simulink model "FourthCOMController"  (Simulink 7.9)
settings: Solver=ode3  StartTime=0.0  StopTime=inf  RelTol=1e-3
libraries: WBCLibrary x10, dspmtrx3 x4, simulink x4, simulink_extras x1
settings Model: Creator=jorhabib  LastModifiedBy=daniele
settings CustomProperty: DataType=string  Value=0

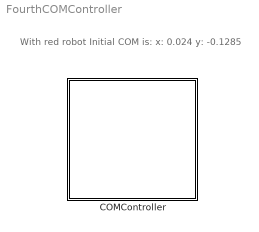
== system FourthCOMController ==
  note: With red robot Initial COM is:
      | x:  0.024
      | y:  -0.1285
  COMController : Subsystem  mask{robotName='icubSim', Ts=0.01}
      mask prompts: robotName "Robot Name"; Ts "Rate (sec)"

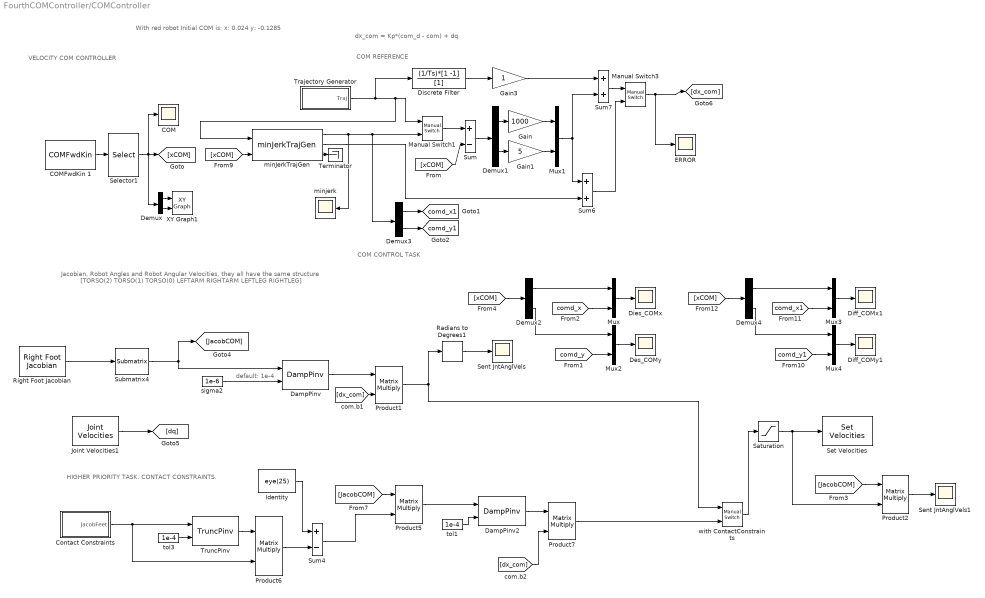
== system FourthCOMController/COMController ==
  note: COM CONTROL TASK
  note: VELOCITY COM CONTROLLER
  note: dx_com = Kp*(com_d - com) + dq
  note: default: 1e-4
  note: Jacobian, Robot Angles and Robot Angular Velocities, they all have the same structure
      | [TORSO(2)  TORSO(1)  TORSO(0)    LEFTARM    RIGHTARM    LEFTLEG    RIGHTLEG]
  note: COM REFERENCE
  note: HIGHER PRIORITY TASK. CONTACT CONSTRAINTS.
  note: With red robot Initial COM is:
      | x:  0.024
      | y:  -0.1285
  COM : Scope
      settings: TimeRange=100  YMin=-0.1  YMax=0.175  SaveName=ScopeData4
  COMFwdKin 1 : WBCLibrary/wholeBodyModel/Forward Kinematics/COMFwdKin   robotName=robotName  localName=localName
  Contact Constraints : Subsystem
  DampPinv : WBCLibrary/Utilities/DampPinv  tol=1e-4
  DampPinv2 : WBCLibrary/Utilities/DampPinv  tol=1e-4
  Demux{,1..4} (5 alike) : Demux  Outputs=2
  Des_COMy : Scope
      settings: TimeRange=100  YMin=-0.1425  YMax=-0.1125  SaveName=ScopeData6
  Dies_COMx : Scope
      settings: TimeRange=100  YMin=0.01  YMax=0.04  SaveName=ScopeData2
  Diff_COMx1 : Scope
      settings: TimeRange=100  YMin=0.0215  YMax=0.03  SaveName=ScopeData5
  Diff_COMy1 : Scope
      settings: TimeRange=100  YMin=-0.135  YMax=-0.0925  SaveName=ScopeData7
  Discrete Filter : DiscreteFilter  Numerator=(1/Ts)*[1 -1]  Denominator=[1]
  ERROR : Scope
      settings: TimeRange=100  YMin=-0.015  YMax=0.015  SaveName=ScopeData3
  Gain : Gain  Gain=1000
  Gain1 : Gain  Gain=5
  Gain3 : Gain
  Identity : Constant  Value=eye(25)
  Joint Velocities1 : WBCLibrary/wholeBodyStates/Joint Velocities  robotName=robotName  localName=localName
  Manual Switch1 : simulink/Signal Routing/Manual Switch  sw=1  action=0  varsize=off
  Manual Switch3 : simulink/Signal Routing/Manual Switch  sw=1  action=0  varsize=off
  Mux{,1..4} (5 alike) : Mux  Inputs=2
  Product{1..2,5..7} (5 alike) : Product  Multiplication=Matrix(*)  RndMeth=Zero
  Radians to Degrees1 : simulink_extras/Transformations/Radians to Degrees
  Right Foot Jacobian : WBCLibrary/wholeBodyModel/Jacobians/Right Foot Jacobian  robotName=robotName  localName=localName
  Saturation : Saturate  UpperLimit=0.8  LowerLimit=-0.8
  Selector1 : Selector  IndexMode=Zero-based  InputPortWidth=7  IndexOptions=Index vector (dialog)  Indices=[0:1]  OutputSizes=1
  Sent JntAnglVels : Scope
      settings: YMin=-0.04  YMax=0.03
  Sent JntAnglVels1 : Scope
      settings: TimeRange=100  YMin=-0.01  YMax=0.01  SaveName=ScopeData8
  Set Velocities : WBCLibrary/wholeBodyActuators/Set Velocities  val=4  robotName=robotName  localName=localName
  Submatrix4 : dspmtrx3/Submatrix  RowSpan=Range of rows  RowStartMode=First  RowStartIndex=1  RowEndMode=Index  RowEndIndex=2  ColSpan=Range of columns  ColStartMode=Index  ColStartIndex=7  ColEndMode=Last  ColEndIndex=6
  Sum : Sum  Inputs=+-
  Sum4 : Sum  Inputs=+-
  Sum6 : Sum
  Sum7 : Sum
  Terminator : Terminator
  Trajectory Generator : Subsystem
  TruncPinv : WBCLibrary/Utilities/TruncPinv  tol=1e-4
  XY Graph1 : simulink/Sinks/XY Graph  xmin=0.01  xmax=0.04  ymin=-0.15  ymax=-0.115  st=-1
  minJerkTrajGen : WBCLibrary/Utilities/minJerkTrajGen  dim=3  Ts=Ts  Tt=Tt
  minjerk : Scope
      settings: TimeRange=100  YMin=-0.12  YMax=-0.025
  sigma2 : Constant  Value=1e-6
  tol1 : Constant  Value=1e-4
  tol3 : Constant  Value=1e-4
  with ContactConstraints : simulink/Signal Routing/Manual Switch  sw=1  action=0  varsize=off
  tag scope: comd_x1=global, comd_y1=global
  wires:
  [xCOM] -> Sum/2
  Sum/1 -> Demux1/1
  Selector1/1 -> [xCOM], Demux/1, COM/1
  COMFwdKin 1/1 -> Selector1/1
  sigma2/1 -> DampPinv/2
  Submatrix4/1 -> DampPinv/1, [JacobCOM]
  [dx_com] -> Product1/2
  Product1/1 -> Radians to Degrees1/1, with ContactConstraints/1
  Radians to Degrees1/1 -> Sent JntAnglVels/1
  Demux/1 -> XY Graph1/1
  Demux/2 -> XY Graph1/2
  Mux/1 -> Dies_COMx/1
  [comd_x] -> Mux/2
  Demux1/1 -> Gain/1
  Demux1/2 -> Gain1/1
  Gain/1 -> Mux1/1
  Gain1/1 -> Mux1/2
  [comd_y] -> Mux2/2
  Mux2/1 -> Des_COMy/1
  [xCOM] -> Demux2/1
  Demux2/1 -> Mux/1
  Demux2/2 -> Mux2/1
  Right Foot Jacobian/1 -> Submatrix4/1
  [JacobCOM] -> Product5/1
  Identity/1 -> Sum4/1
  tol3/1 -> TruncPinv/2
  TruncPinv/1 -> Product6/1
  Product6/1 -> Sum4/2
  Contact Constraints/1(JacobFeet) -> TruncPinv/1, Product6/2
  Sum4/1 -> Product5/2
  Product5/1 -> DampPinv2/1
  tol1/1 -> DampPinv2/2
  [dx_com] -> Product7/2
  Product7/1 -> with ContactConstraints/2
  with ContactConstraints/1 -> Saturation/1
  Manual Switch1/1 -> Sum/1
  Trajectory Generator/1(Traj) -> minJerkTrajGen/1, Manual Switch1/1, Discrete Filter/1
  [xCOM] -> minJerkTrajGen/2
  minJerkTrajGen/1 -> minjerk/1, Manual Switch1/2, Demux3/1
  Mux1/1 -> Sum6/1, Sum7/2
  Sum6/1 -> Manual Switch3/2
  minJerkTrajGen/2 -> Sum6/2
  Demux3/1 -> [comd_x1]
  Demux3/2 -> [comd_y1]
  Mux3/1 -> Diff_COMx1/1
  [comd_x1] -> Mux3/2
  [comd_y1] -> Mux4/2
  Mux4/1 -> Diff_COMy1/1
  [xCOM] -> Demux4/1
  Demux4/1 -> Mux3/1
  Demux4/2 -> Mux4/1
  Discrete Filter/1 -> Gain3/1
  Sum7/1 -> Manual Switch3/1
  Manual Switch3/1 -> [dx_com], ERROR/1
  Gain3/1 -> Sum7/1
  Saturation/1 -> Set Velocities/1, Product2/2
  [JacobCOM] -> Product2/1
  Product2/1 -> Sent JntAnglVels1/1
  DampPinv/1 -> Product1/1
  DampPinv2/1 -> Product7/1
  Joint Velocities1/1 -> [dq]
  minJerkTrajGen/3 -> Terminator/1

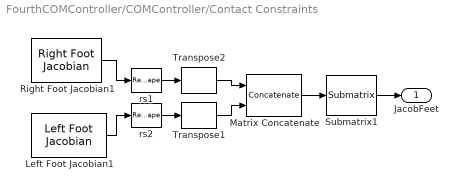
== system FourthCOMController/COMController/Contact Constraints ==
  Left Foot Jacobian1 : WBCLibrary/wholeBodyModel/Jacobians/Left Foot Jacobian  robotName=robotName  localName=localName
  Matrix Concatenate : Concatenate  Mode=Multidimensional array
  Right Foot Jacobian1 : WBCLibrary/wholeBodyModel/Jacobians/Right Foot Jacobian  robotName=robotName  localName=localName
  Submatrix1 : dspmtrx3/Submatrix  RowSpan=Range of rows  RowStartMode=First  RowStartIndex=1  RowEndMode=Index  RowEndIndex=2  ColSpan=Range of columns  ColStartMode=Index  ColStartIndex=7  ColEndMode=Last  ColEndIndex=6
  Transpose1 : dspmtrx3/Transpose  Hermitian=off  overflowFlag=off
  Transpose2 : dspmtrx3/Transpose  Hermitian=off  overflowFlag=off
  rs1 : Reshape  OutputDimensionality=Customize  OutputDimensions=[31,6]
  rs2 : Reshape  OutputDimensionality=Customize  OutputDimensions=[31,6]
  JacobFeet : Outport
  wires:
  Right Foot Jacobian1/1 -> rs1/1
  Left Foot Jacobian1/1 -> rs2/1
  rs1/1 -> Transpose2/1
  rs2/1 -> Transpose1/1
  Transpose2/1 -> Matrix Concatenate/1
  Transpose1/1 -> Matrix Concatenate/2
  Matrix Concatenate/1 -> Submatrix1/1
  Submatrix1/1 -> JacobFeet/1

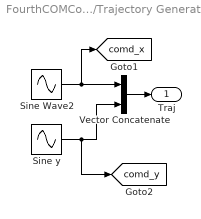
== system FourthCOMController/COMController/Trajectory Generator ==
  Sine Wave2 : Sin  Amplitude=0.01  Bias=0.02407  Frequency=0.2  Phase=pi/2
  Sine y : Sin  Amplitude=0.01  Bias=-0.1287  Frequency=0.2
  Vector Concatenate : Concatenate
  Traj : Outport
  tag scope: comd_x=global, comd_y=global
  wires:
  Sine Wave2/1 -> Vector Concatenate/1, [comd_x]
  Sine y/1 -> Vector Concatenate/2, [comd_y]
  Vector Concatenate/1 -> Traj/1
